simulink model "robust_proximity_sliding_mode"  (R2019b)
settings: Solver=VariableStepAuto  StartTime=0.0  StopTime=10.0  RelTol=1e-3
settings Model: Creator=Alien  LastModifiedBy=Alien

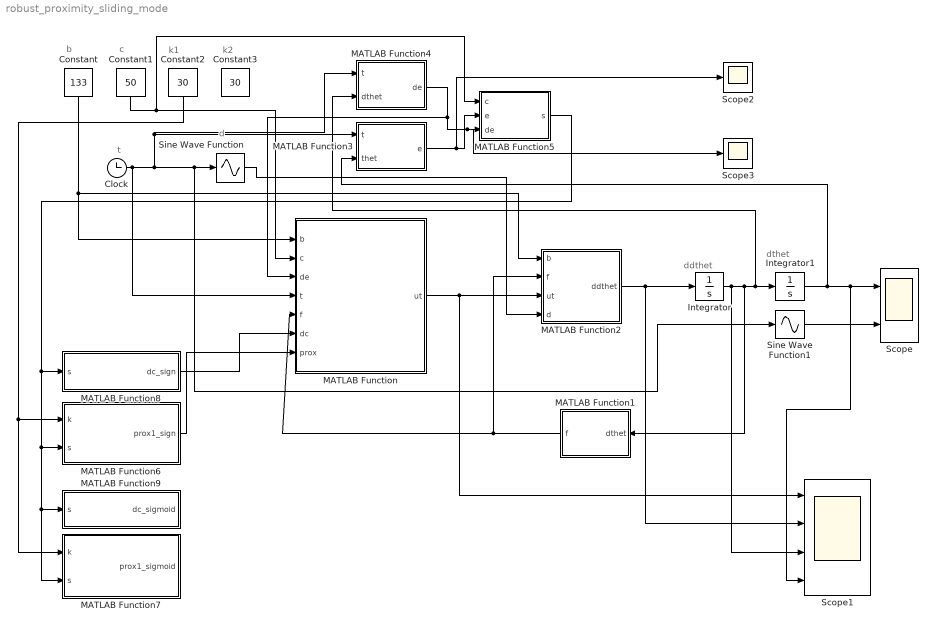
== system robust_proximity_sliding_mode ==
  note: k2
  note: k1
  note: c
  note: b
  note: d
  note: t
  note: ddthet
  note: dthet
  Clock : Clock
  Constant : Constant  Value=133
  Constant1 : Constant  Value=50
  Constant2 : Constant  Value=30
  Constant3 : Constant  Value=30
  Integrator : Integrator  InitialCondition=5
  Integrator1 : Integrator  InitialCondition=2
  MATLAB Function : MATLAB Function  TreatAsAtomicUnit=on
  MATLAB Function1 : MATLAB Function  TreatAsAtomicUnit=on
  MATLAB Function2 : MATLAB Function  TreatAsAtomicUnit=on
  MATLAB Function3 : MATLAB Function  TreatAsAtomicUnit=on
  MATLAB Function4 : MATLAB Function  TreatAsAtomicUnit=on
  MATLAB Function5 : MATLAB Function  TreatAsAtomicUnit=on
  MATLAB Function6 : MATLAB Function  TreatAsAtomicUnit=on
  MATLAB Function7 : MATLAB Function  TreatAsAtomicUnit=on
  MATLAB Function8 : MATLAB Function  TreatAsAtomicUnit=on
  MATLAB Function9 : MATLAB Function  TreatAsAtomicUnit=on
  Scope : Scope  NumInputPorts=2
  Scope1 : Scope  NumInputPorts=4
  Scope2 : Scope
  Scope3 : Scope
  Sine Wave Function : Sin  TimeSource=Use external signal  Amplitude=10  Frequency=pi  SampleTime=0
  Sine Wave Function1 : Sin  TimeSource=Use external signal  SampleTime=0
  wires:
  Integrator/1 -> Scope1/3, MATLAB Function1/1(dthet), MATLAB Function4/2(dthet), Integrator1/1
  Clock/1 -> MATLAB Function/4(t), MATLAB Function3/1(t), MATLAB Function4/1(t), Sine Wave Function1/1, Sine Wave Function/1
  MATLAB Function2/1(ddthet) -> Scope1/2, Integrator/1
  MATLAB Function5/1(s) -> MATLAB Function7/2(s), MATLAB Function9/1(s), MATLAB Function6/2(s), MATLAB Function8/1(s)
  Constant2/1 -> MATLAB Function7/1(k), MATLAB Function6/1(k)
  MATLAB Function1/1(f) -> MATLAB Function2/2(f), MATLAB Function/5(f)
  MATLAB Function/1(ut) -> Scope1/1, MATLAB Function2/3(ut)
  Constant/1 -> MATLAB Function2/1(b), MATLAB Function/1(b)
  Constant1/1 -> MATLAB Function5/1(c), MATLAB Function/2(c)
  MATLAB Function4/1(de) -> Scope3/1, MATLAB Function5/3(de), MATLAB Function/3(de)
  MATLAB Function3/1(e) -> Scope2/1, MATLAB Function5/2(e)
  Integrator1/1 -> Scope1/4, Scope/1, MATLAB Function3/2(thet)
  Sine Wave Function/1 -> MATLAB Function2/4(d)
  Sine Wave Function1/1 -> Scope/2
  MATLAB Function6/1(prox1_sign) -> MATLAB Function/7(prox)
  MATLAB Function8/1(dc_sign) -> MATLAB Function/6(dc)

== matlab function robust_proximity_sliding_mode/MATLAB Function1 ==
  data: dthet input; f output
function f = fcn(dthet)
f = 25*dthet;

== matlab function robust_proximity_sliding_mode/MATLAB Function ==
  data: b input; ut output; c input; de input; t input; f input; dc input; prox input
function ut = fcn(b, c, de, t, f, dc, prox)
ddthet_d = -sin(t);
ut = 1 / b * (c * de +ddthet_d + f - dc - prox);

== matlab function robust_proximity_sliding_mode/MATLAB Function2 ==
  data: b input; ddthet output; f input; ut input; d input
function ddthet = fcn(b, f, ut, d)
ddthet = b * ut - f + d;

== matlab function robust_proximity_sliding_mode/MATLAB Function3 ==
  data: t input; e output; thet input
function e = fcn(t, thet)
e = sin(t) - thet;

== matlab function robust_proximity_sliding_mode/MATLAB Function4 ==
  data: t input; de output; dthet input
function de = fcn(t, dthet)
de = cos(t) - dthet;

== matlab function robust_proximity_sliding_mode/MATLAB Function5 ==
  data: c input; s output; e input; de input
function s = fcn(c, e, de)
s = c * e + de;

== matlab function robust_proximity_sliding_mode/MATLAB Function6 ==
  data: k input; prox1_sign output; s input
function prox1_sign= fcn(k, s)
sigma = 0.5;
prox1_sign = (-1)* k * s - sigma * sign(s);

== matlab function robust_proximity_sliding_mode/MATLAB Function7 ==
  data: k input; prox1_sigmoid output; s input
function prox1_sigmoid = fcn(k, s)
sigma = 0.5;
sigmoid =1./(1+exp(-s));
prox1_sigmoid = (-1)* k * s - sigma * sigmoid;

== matlab function robust_proximity_sliding_mode/MATLAB Function8 ==
  data: s input; dc_sign output
function dc_sign = fcn(s)
du = 10;
dl = -10;
d1 = (du - dl)/2;
d2 = (du + dl)/2;
dc_sign = d2 - d1 * sign(s);

== matlab function robust_proximity_sliding_mode/MATLAB Function9 ==
  data: s input; dc_sigmoid output
function dc_sigmoid = fcn(s)
du = 10;
dl = -10;
d1 = (du - dl)/2;
d2 = (du + dl)/2;
sigmoid =1./(1+exp(-s));
dc_sigmoid = d2 - d1 * sigmoid;
